simulink model "im_foc_models_digital"  (R2022b)
settings: Solver=VariableStepAuto  StartTime=0.0  StopTime=2  FixedStep=0.00001  RelTol=1e-3
undefined symbols (not defined in the file or in its folder): B, J, K1, K2, K3, K4, K5, K6, K7, K8, K9, Lm, Lr, Lsigma, pole, sigbuilder_block
settings Model: Creator=jack  LastModifiedBy=jack

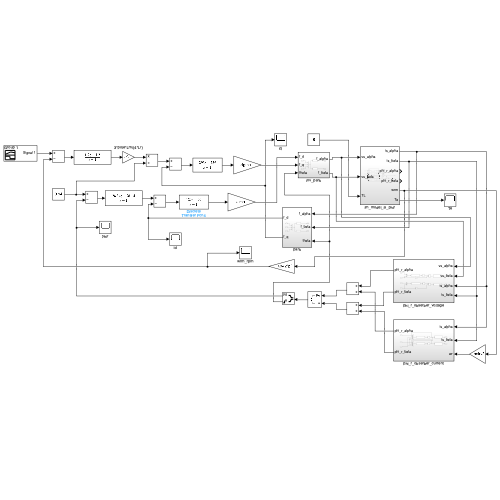
[thumbnail: Simulink's stored preview of the top-level diagram]
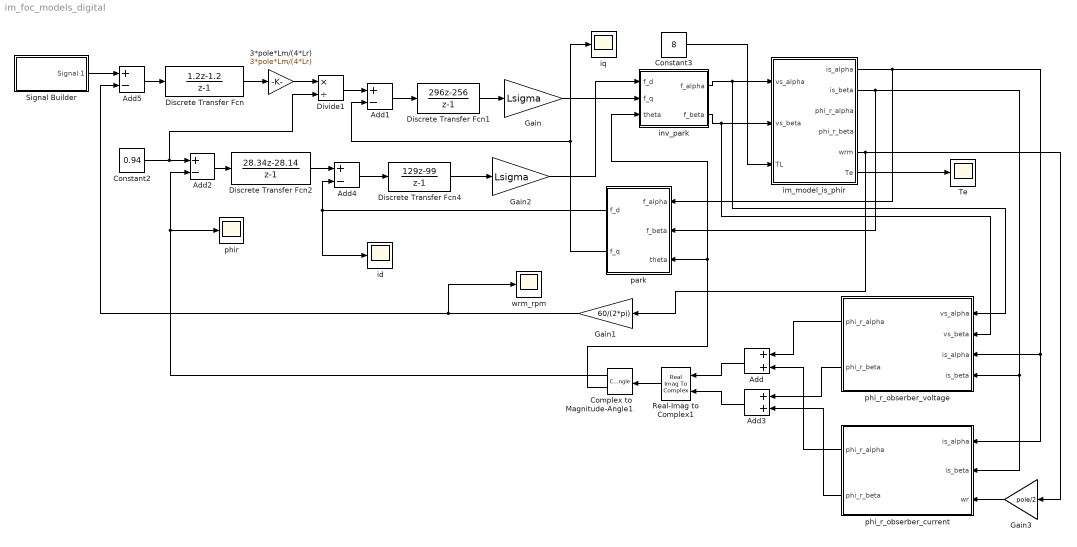
== system im_foc_models_digital ==
  3*pole*Lm/(4*Lr) : Gain  Gain=3*pole*Lm/(4*Lr)
  Add : Sum
  Add{1..2,4..5} (4 alike) : Sum  Inputs=+-
  Add3 : Sum
  Complex to Magnitude-Angle1 : ComplexToMagnitudeAngle
  Constant2 : Constant  Value=0.94
  Constant3 : Constant  Value=8
  Discrete Transfer Fcn : DiscreteTransferFcn  Numerator=[1.2 -1.2]  Denominator=[1 -1]  SampleTime=0.001
  Discrete Transfer Fcn1 : DiscreteTransferFcn  Numerator=[296 -256]  Denominator=[1 -1]  SampleTime=0.001
  Discrete Transfer Fcn2 : DiscreteTransferFcn  Numerator=[28.34 -28.14]  Denominator=[1 -1]  SampleTime=0.001
  Discrete Transfer Fcn4 : DiscreteTransferFcn  Numerator=[129 -99]  Denominator=[1 -1]  SampleTime=0.001
  Divide1 : Product  Inputs=*/
  Gain : Gain  Gain=Lsigma
  Gain1 : Gain  Gain=60/(2*pi)
  Gain2 : Gain  Gain=Lsigma
  Gain3 : Gain  Gain=pole/2
  Real-Imag to Complex1 : RealImagToComplex
  Signal Builder : Subsystem  Tag=STV Subsys  LoadFcn=sigbuilder_block('load');  StartFcn=sigbuilder_block('start');  StopFcn=sigbuilder_block('stop');  ClipboardFcn=sigbuilder_block('clipboard');  mask(Sigbuilder block){tuvar=[0:10]}
      mask help: Simulink:masks:SigbuilderBlock_MD
      mask init:
      | if ~strcmp(get_param(bdroot(gcbh),'SimulationStatus'),'stopped') tuvar = sigbuilder_block('maskInit'); end
      settings: CopyFcn=sigbuilder_block('copy');  DeleteFcn=sigbuilder_block('delete');  ModelCloseFcn=sigbuilder_block('modelClose');  PreSaveFcn=sigbuilder_block('preSave');  PauseFcn=sigbuilder_block('pause');  ContinueFcn=sigbuilder_block('continue');  NameChangeFcn=sigbuilder_block('namechange');  OpenFcn=sigbuilder_block('open',[346 178 550 400 ]);  CloseFcn=sigbuilder_block('close');
      mask Display: plot(0, 0, 100, 100,[2, 2, 32, 32, 2], [68, 8, 8, 68, 68],[32, 2], [38, 38], [32, 19, 2],[53, 60, 44], [32, 17, 17, 2],[16, 16, 31, 31]);txt = getActiveGroup(gcbh);text(2, 100, txt,'verticalAlignment', 'top');
  Te : Scope
  id : Scope
  im_model_is_phir : Subsystem
  inv_park : Subsystem
  iq : Scope
  park : Subsystem
  phi_r_obserber_current : Subsystem
  phi_r_obserber_voltage : Subsystem
  phir : Scope
  wrm_rpm : Scope
  wires:
  Discrete Transfer Fcn/1 -> 3*pole*Lm/(4*Lr)/1
  3*pole*Lm/(4*Lr)/1 -> Divide1/1
  Constant2/1 -> Divide1/2, Add2/1
  Divide1/1 -> Add1/1
  Add1/1 -> Discrete Transfer Fcn1/1
  Add2/1 -> Discrete Transfer Fcn2/1
  Discrete Transfer Fcn2/1 -> Add4/1
  Add4/1 -> Discrete Transfer Fcn4/1
  Discrete Transfer Fcn4/1 -> Gain2/1
  Add5/1 -> Discrete Transfer Fcn/1
  Signal Builder/1(Signal 1) -> Add5/1
  Gain1/1 -> wrm_rpm/1, Add5/2
  Gain/1 -> inv_park/2(f_q)
  inv_park/1(f_alpha) -> phi_r_obserber_voltage/1(vs_alpha), im_model_is_phir/1(vs_alpha)
  inv_park/2(f_beta) -> phi_r_obserber_voltage/2(vs_beta), im_model_is_phir/2(vs_beta)
  Constant3/1 -> im_model_is_phir/3(TL)
  im_model_is_phir/5(wrm) -> Gain3/1, Gain1/1
  im_model_is_phir/1(is_alpha) -> park/1(f_alpha), phi_r_obserber_voltage/3(is_alpha), phi_r_obserber_current/1(is_alpha)
  im_model_is_phir/2(is_beta) -> park/2(f_beta), phi_r_obserber_voltage/4(is_beta), phi_r_obserber_current/2(is_beta)
  Discrete Transfer Fcn1/1 -> Gain/1
  park/2(f_q) -> Add1/2, iq/1
  park/1(f_d) -> id/1, Add4/2
  Gain2/1 -> inv_park/1(f_d)
  im_model_is_phir/6(Te) -> Te/1
  Real-Imag to Complex1/1 -> Complex to Magnitude-Angle1/1
  Complex to Magnitude-Angle1/1 -> Add2/2, phir/1
  Complex to Magnitude-Angle1/2 -> inv_park/3(theta), park/3(theta)
  Gain3/1 -> phi_r_obserber_current/3(wr)
  phi_r_obserber_voltage/1(phi_r_alpha) -> Add/1
  phi_r_obserber_current/1(phi_r_alpha) -> Add/2
  phi_r_obserber_voltage/2(phi_r_beta) -> Add3/1
  phi_r_obserber_current/2(phi_r_beta) -> Add3/2
  Add/1 -> Real-Imag to Complex1/1
  Add3/1 -> Real-Imag to Complex1/2

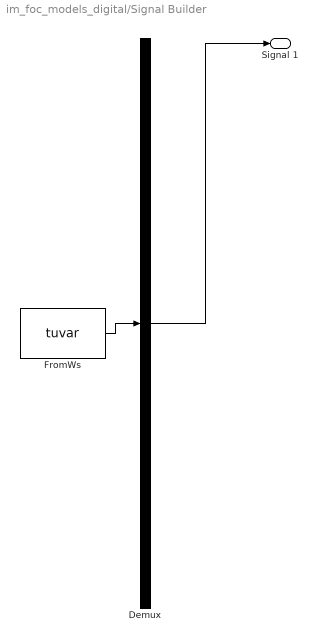
== system im_foc_models_digital/Signal Builder ==
  Demux : Demux  Tag=STV Demux  Outputs=1
      settings: DisplayOption=none
  FromWs : FromWorkspace  Tag=STV FromWs  VariableName=tuvar
      SigBuilderData=|
      | common.afterFinalStr = 'Extrapolate'
      | common.sampleTime = 0
      | dataSet.timeRange = [0 10]
      | dataSet.name = 'Group 1'
      | sbobj.Groups.Name = 'Group 1'
      | sbobj.Groups.Signals.Name = 'Signal 1'
      | sbobj.Groups.Signals.XData = [0 1 4 6 10]
      | sbobj.Groups.Signals.YData = [0 1000 1000 1000 1000]
  Signal 1 : Outport  Tag=STV Outport
  wires:
  Demux/1 -> Signal 1/1
  FromWs/1 -> Demux/1

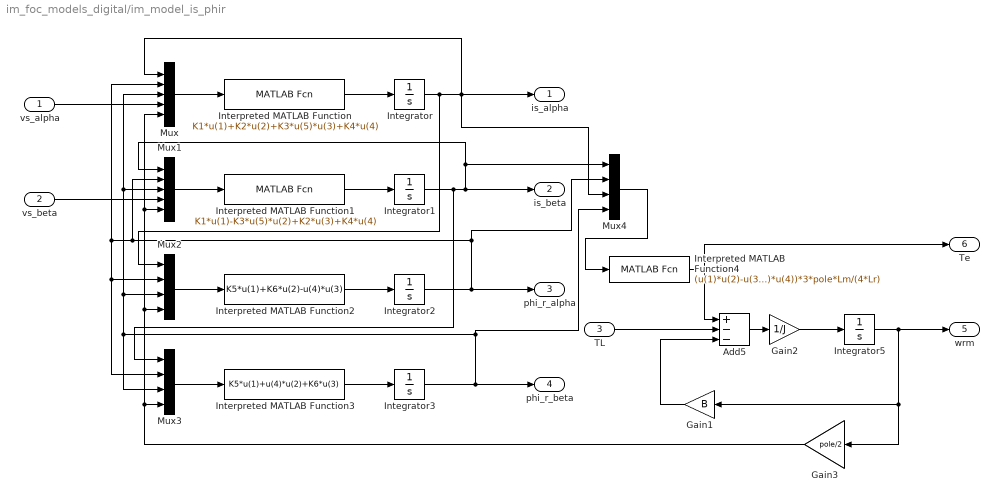
== system im_foc_models_digital/im_model_is_phir ==
  vs_alpha : Inport
  vs_beta : Inport  Port=2
  TL : Inport  Port=3
  Add5 : Sum  Inputs=+--
  Gain1 : Gain  Gain=B
  Gain2 : Gain  Gain=1/J
  Gain3 : Gain  Gain=pole/2
  Integrator{,1..3,5} (5 alike) : Integrator
  Interpreted MATLAB Function : MATLABFcn  MATLABFcn=K1*u(1)+K2*u(2)+K3*u(5)*u(3)+K4*u(4)
  Interpreted MATLAB Function1 : MATLABFcn  MATLABFcn=K1*u(1)-K3*u(5)*u(2)+K2*u(3)+K4*u(4)
  Interpreted MATLAB Function2 : MATLABFcn  MATLABFcn=K5*u(1)+K6*u(2)-u(4)*u(3)
  Interpreted MATLAB Function3 : MATLABFcn  MATLABFcn=K5*u(1)+u(4)*u(2)+K6*u(3)
  Interpreted MATLAB Function4 : MATLABFcn  MATLABFcn=(u(1)*u(2)-u(3)*u(4))*3*pole*Lm/(4*Lr)
  Mux : Mux  Inputs=5
  Mux1 : Mux  Inputs=5
  Mux2 : Mux
  Mux3 : Mux
  Mux4 : Mux
  is_alpha : Outport
  is_beta : Outport  Port=2
  phi_r_alpha : Outport  Port=3
  phi_r_beta : Outport  Port=4
  wrm : Outport  Port=5
  Te : Outport  Port=6
  wires:
  Add5/1 -> Gain2/1
  Interpreted MATLAB Function2/1 -> Integrator2/1
  vs_beta/1 -> Mux1/4
  vs_alpha/1 -> Mux/4
  Mux3/1 -> Interpreted MATLAB Function3/1
  Interpreted MATLAB Function1/1 -> Integrator1/1
  Mux4/1 -> Interpreted MATLAB Function4/1
  Integrator1/1 -> Mux3/1, is_beta/1, Mux1/1, Mux4/1
  Gain1/1 -> Add5/3
  TL/1 -> Add5/2
  Interpreted MATLAB Function4/1 -> Te/1, Add5/1
  Integrator5/1 -> wrm/1, Gain1/1, Gain3/1
  Integrator2/1 -> phi_r_alpha/1, Mux4/2, Mux1/2, Mux/2, Mux3/2, Mux2/2
  Integrator3/1 -> phi_r_beta/1, Mux4/4, Mux3/3, Mux2/3, Mux/3, Mux1/3
  Mux1/1 -> Interpreted MATLAB Function1/1
  Interpreted MATLAB Function3/1 -> Integrator3/1
  Mux2/1 -> Interpreted MATLAB Function2/1
  Mux/1 -> Interpreted MATLAB Function/1
  Gain2/1 -> Integrator5/1
  Interpreted MATLAB Function/1 -> Integrator/1
  Integrator/1 -> Mux2/1, is_alpha/1, Mux4/3, Mux/1
  Gain3/1 -> Mux3/4, Mux2/4, Mux1/5, Mux/5

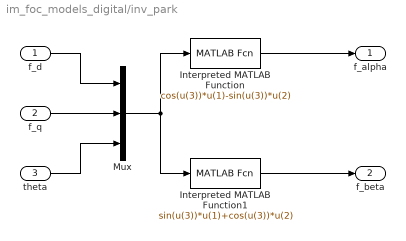
== system im_foc_models_digital/inv_park ==
  f_d : Inport
  f_q : Inport  Port=2
  theta : Inport  Port=3
  Interpreted MATLAB Function : MATLABFcn  MATLABFcn=cos(u(3))*u(1)-sin(u(3))*u(2)
  Interpreted MATLAB Function1 : MATLABFcn  MATLABFcn=sin(u(3))*u(1)+cos(u(3))*u(2)
  Mux : Mux  Inputs=3
  f_alpha : Outport
  f_beta : Outport  Port=2
  wires:
  Interpreted MATLAB Function/1 -> f_alpha/1
  f_d/1 -> Mux/1
  Mux/1 -> Interpreted MATLAB Function1/1, Interpreted MATLAB Function/1
  Interpreted MATLAB Function1/1 -> f_beta/1
  theta/1 -> Mux/3
  f_q/1 -> Mux/2

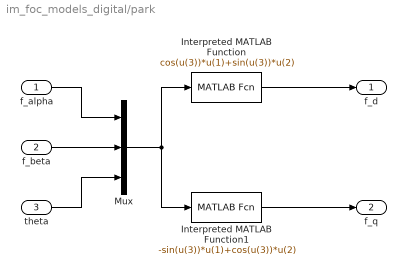
== system im_foc_models_digital/park ==
  f_alpha : Inport
  f_beta : Inport  Port=2
  theta : Inport  Port=3
  Interpreted MATLAB Function : MATLABFcn  MATLABFcn=cos(u(3))*u(1)+sin(u(3))*u(2)
  Interpreted MATLAB Function1 : MATLABFcn  MATLABFcn=-sin(u(3))*u(1)+cos(u(3))*u(2)
  Mux : Mux  Inputs=3
  f_d : Outport
  f_q : Outport  Port=2
  wires:
  Interpreted MATLAB Function/1 -> f_d/1
  f_alpha/1 -> Mux/1
  Mux/1 -> Interpreted MATLAB Function1/1, Interpreted MATLAB Function/1
  Interpreted MATLAB Function1/1 -> f_q/1
  theta/1 -> Mux/3
  f_beta/1 -> Mux/2

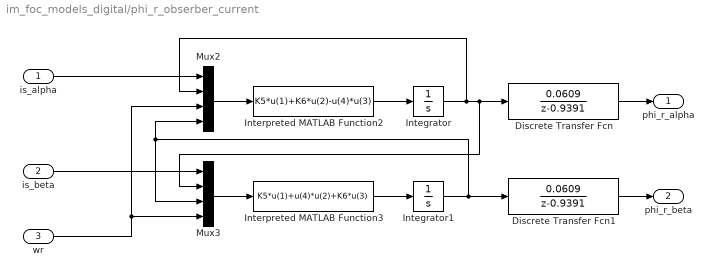
== system im_foc_models_digital/phi_r_obserber_current ==
  is_alpha : Inport
  is_beta : Inport  Port=2
  wr : Inport  Port=3
  Discrete Transfer Fcn : DiscreteTransferFcn  Numerator=[0.0609]  Denominator=[1 -0.9391]  SampleTime=0.001
  Discrete Transfer Fcn1 : DiscreteTransferFcn  Numerator=[0.0609]  Denominator=[1 -0.9391]  SampleTime=0.001
  Integrator : Integrator
  Integrator1 : Integrator
  Interpreted MATLAB Function2 : MATLABFcn  MATLABFcn=K5*u(1)+K6*u(2)-u(4)*u(3)
  Interpreted MATLAB Function3 : MATLABFcn  MATLABFcn=K5*u(1)+u(4)*u(2)+K6*u(3)
  Mux2 : Mux
  Mux3 : Mux
  phi_r_alpha : Outport
  phi_r_beta : Outport  Port=2
  wires:
  is_beta/1 -> Mux3/1
  wr/1 -> Mux3/4, Mux2/3
  is_alpha/1 -> Mux2/1
  Mux2/1 -> Interpreted MATLAB Function2/1
  Integrator1/1 -> Discrete Transfer Fcn1/1, Mux3/3, Mux2/4
  Integrator/1 -> Discrete Transfer Fcn/1, Mux3/2, Mux2/2
  Interpreted MATLAB Function2/1 -> Integrator/1
  Mux3/1 -> Interpreted MATLAB Function3/1
  Interpreted MATLAB Function3/1 -> Integrator1/1
  Discrete Transfer Fcn/1 -> phi_r_alpha/1
  Discrete Transfer Fcn1/1 -> phi_r_beta/1

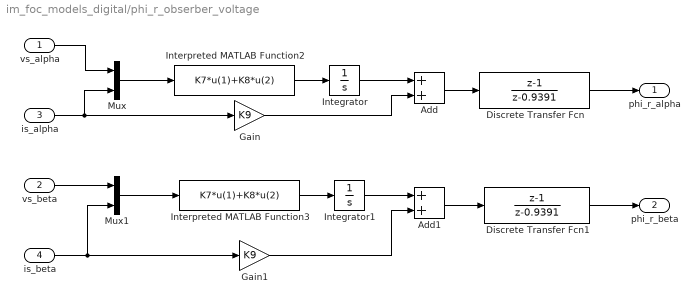
== system im_foc_models_digital/phi_r_obserber_voltage ==
  vs_alpha : Inport
  vs_beta : Inport  Port=2
  is_alpha : Inport  Port=3
  is_beta : Inport  Port=4
  Add : Sum
  Add1 : Sum
  Discrete Transfer Fcn : DiscreteTransferFcn  Numerator=[1 -1]  Denominator=[1 -0.9391]  SampleTime=0.001
  Discrete Transfer Fcn1 : DiscreteTransferFcn  Numerator=[1 -1]  Denominator=[1 -0.9391]  SampleTime=0.001
  Gain : Gain  Gain=K9
  Gain1 : Gain  Gain=K9
  Integrator : Integrator
  Integrator1 : Integrator
  Interpreted MATLAB Function2 : MATLABFcn  MATLABFcn=K7*u(1)+K8*u(2)
  Interpreted MATLAB Function3 : MATLABFcn  MATLABFcn=K7*u(1)+K8*u(2)
  Mux : Mux  Inputs=2
  Mux1 : Mux  Inputs=2
  phi_r_alpha : Outport
  phi_r_beta : Outport  Port=2
  wires:
  Interpreted MATLAB Function2/1 -> Integrator/1
  Interpreted MATLAB Function3/1 -> Integrator1/1
  vs_alpha/1 -> Mux/1
  is_alpha/1 -> Gain/1, Mux/2
  Mux/1 -> Interpreted MATLAB Function2/1
  Integrator/1 -> Add/1
  Add/1 -> Discrete Transfer Fcn/1
  Gain/1 -> Add/2
  Integrator1/1 -> Add1/1
  Add1/1 -> Discrete Transfer Fcn1/1
  is_beta/1 -> Mux1/2, Gain1/1
  vs_beta/1 -> Mux1/1
  Mux1/1 -> Interpreted MATLAB Function3/1
  Gain1/1 -> Add1/2
  Discrete Transfer Fcn/1 -> phi_r_alpha/1
  Discrete Transfer Fcn1/1 -> phi_r_beta/1
